simulink model "PDcontroller"  (Simulink 7.5)
settings: Solver=ode15s  StartTime=0.0  StopTime=10  FixedStep=1  RelTol=1e-3
undefined symbols (not defined in the file or in its folder): Cmat_sim, Dmat_sim, Gmat_sim
settings Model: Creator=Prasad  LastModifiedBy=Prasad
settings SimEventsCC: propDiagAttribOutput=1  propDiagFcnCallOutput=1  propDiagStatOutput=0

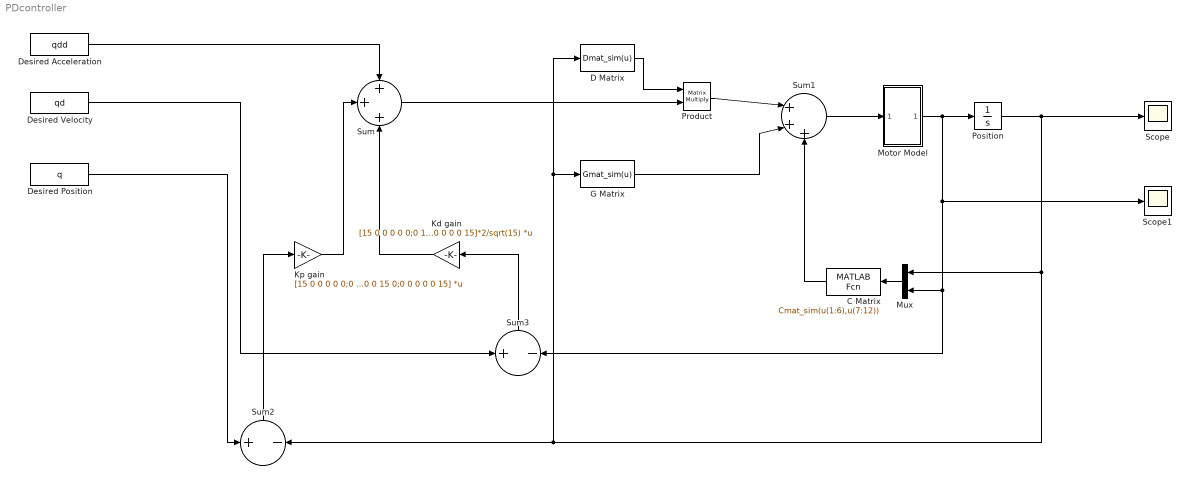
== system PDcontroller ==
  C Matrix : MATLABFcn  MATLABFcn=Cmat_sim(u(1:6),u(7:12))  OutputDimensions=[6 1]  OutputSignalType=real  Output1D=off
  D Matrix : MATLABFcn  MATLABFcn=Dmat_sim(u)  OutputSignalType=real  Output1D=off
  Desired Acceleration : FromWorkspace  VariableName=qdd  SampleTime=0  OutputAfterFinalValue=Holding final value
  Desired Position : FromWorkspace  VariableName=q  SampleTime=0  OutputAfterFinalValue=Holding final value
  Desired Velocity : FromWorkspace  VariableName=qd  SampleTime=0  OutputAfterFinalValue=Holding final value
  G Matrix : MATLABFcn  MATLABFcn=Gmat_sim(u)  OutputSignalType=real  Output1D=off
  Kd gain : Gain  Gain=[15 0 0 0 0 0;0 15 0 0 0 0;0 0 3 0 0 0;0 0 0 15 0 0;0 0 0 0 15 0;0 0 0 0 0 15]*2/sqrt(15)  Multiplication=Matrix(K*u)  ParameterDataType=fixdt(1, 16)  ParameterScaling=2^0  OutDataType=fixdt(1, 16)  OutScaling=2^0
  Kp gain : Gain  Gain=[15 0 0 0 0 0;0 15 0 0 0 0;0 0 35 0 0 0;0 0 0 15 0 0;0 0 0 0 15 0;0 0 0 0 0 15]  Multiplication=Matrix(K*u)  ParameterDataType=fixdt(1, 16)  ParameterScaling=2^0  OutDataType=fixdt(1, 16)  OutScaling=2^0
  Motor Model : Subsystem
  Mux : Mux  Inputs=2
  Position : Integrator  InitialCondition=[1 1 1 1 1 1]
  Product : Product  Multiplication=Matrix(*)  OutDataType=fixdt(1, 16)  OutScaling=2^0  RndMeth=Zero
  Scope : Scope
      settings: TimeRange=20  YMin=-1  YMax=4
  Scope1 : Scope
      settings: TimeRange=20  YMin=-1  YMax=4
  Sum : Sum  Inputs=+++  OutDataType=fixdt(1, 16)  OutScaling=2^0
  Sum1 : Sum  Inputs=|+++  OutDataType=fixdt(1, 16)  OutScaling=2^0
  Sum2 : Sum  Inputs=+|-  OutDataType=fixdt(1, 16)  OutScaling=2^0
  Sum3 : Sum  Inputs=+-  OutDataType=fixdt(1, 16)  OutScaling=2^0
  wires:
  D Matrix/1 -> Product/1
  G Matrix/1 -> Sum1/2
  Product/1 -> Sum1/1
  C Matrix/1 -> Sum1/3
  Sum/1 -> Product/2
  Sum1/1 -> Motor Model/1(In1)
  Motor Model/1(Out1) -> Position/1, Sum3/2, Mux/2, Scope1/1
  Position/1 -> Mux/1, Sum2/2, D Matrix/1, G Matrix/1, Scope/1
  Mux/1 -> C Matrix/1
  Desired Acceleration/1 -> Sum/1
  Desired Velocity/1 -> Sum3/1
  Desired Position/1 -> Sum2/1
  Kp gain/1 -> Sum/2
  Sum2/1 -> Kp gain/1
  Sum3/1 -> Kd gain/1
  Kd gain/1 -> Sum/3

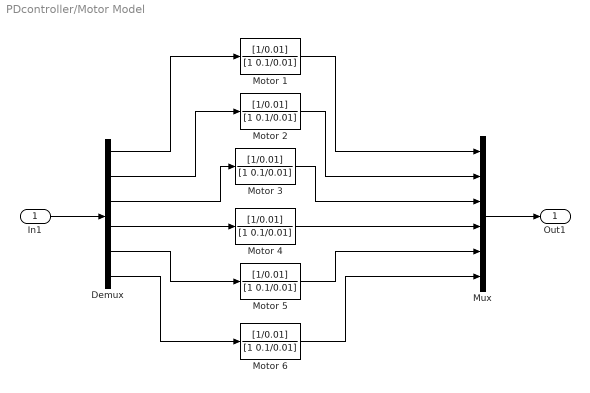
== system PDcontroller/Motor Model ==
  In1 : Inport
  Demux : Demux  Outputs=6
  Motor {1..6} (6 alike) : TransferFcn  Numerator=[1/0.01]  Denominator=[1 0.1/0.01]
  Mux : Mux  Inputs=6
  Out1 : Outport
  wires:
  Mux/1 -> Out1/1
  Motor 6/1 -> Mux/6
  Motor 5/1 -> Mux/5
  Motor 4/1 -> Mux/4
  Motor 3/1 -> Mux/3
  Motor 2/1 -> Mux/2
  Motor 1/1 -> Mux/1
  Demux/6 -> Motor 6/1
  Demux/5 -> Motor 5/1
  Demux/4 -> Motor 4/1
  Demux/3 -> Motor 3/1
  Demux/2 -> Motor 2/1
  Demux/1 -> Motor 1/1
  In1/1 -> Demux/1
